simulink model "Simulacao_Exemplo_2B"  (R2020a)
settings: Solver=ode45  StartTime=0.0  StopTime=240  FixedStep=0.1  MaxStep=5e-1  RelTol=1e-3  EnableMultiTasking=on
settings Model: Creator=MeneghettiAir  LastModifiedBy=jhona
settings DataIOCC: LimitDataPoints=on  SaveFormat=Array  ReturnWorkspaceOutputs=off
settings OptimizationCC: LifeSpan=inf
settings DebuggingCC: SolverPrmCheckMsg=warning  SFUnexpectedBacktrackingDiag=warning  SFNoUnconditionalDefaultTransitionDiag=warning  SFExecutionAtInitializationDiag=none  ArithmeticOperatorsInVariantConditions=warning
settings HardwareCC: ProdBitPerPointer=32  ProdBitPerSizeT=32  ProdBitPerPtrDiffT=32  ProdLargestAtomicFloat=None  ProdIntDivRoundTo=Undefined  ProdEndianess=Unspecified  ProdWordSize=32  ProdHWDeviceType=32-bit Generic
settings ModelReferenceCC: PropagateSignalLabelsOutOfModel=off
settings SFSimCC: SimUseLocalCustomCode=off  CustomCodeUndefinedFunction=UseInterfaceOnly
settings RTWCC: RTWUseLocalCustomCode=off
settings CodeAppCC: StateflowObjectComments=on
settings GRTTargetCC: TargetLangStandard=C89/C90 (ANSI)
settings ConfigComp: CovMetricSettings=dw  CovHtmlReporting=on  CovSaveCumulativeToWorkspaceVar=on  CovSaveSingleToWorkspaceVar=on  CovExternalEMLEnable=off  CovSFcnEnable=off

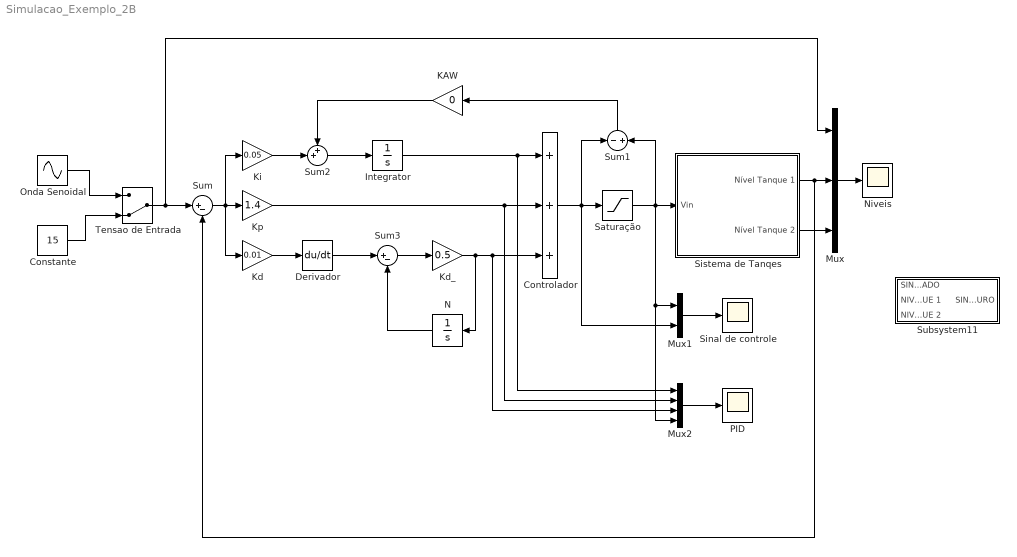
== system Simulacao_Exemplo_2B ==
  Constante : Constant  Value=15
  Controlador : Sum  Inputs=+++
  Derivador : Derivative
  Integrator : Integrator
  KAW : Gain  Gain=0
  Kd : Gain  Gain=0.01
  Kd_ : Gain  Gain=0.5
  Ki : Gain  Gain=0.05
  Kp : Gain  Gain=1.4
  Mux : Mux  Inputs=3
  Mux1 : Mux  Inputs=2
  Mux2 : Mux
  N : Integrator
  Niveis : Scope
  Onda Senoidal : Sin  Amplitude=2  Bias=14  Frequency=0.2  SampleTime=0
  PID : Scope
  Saturação : Saturate  UpperLimit=4  LowerLimit=-4
  Sinal de controle : Scope
  "Sistema de Tanqes " : Subsystem
  Subsystem11 : Subsystem
  Sum : Sum  Inputs=|+-
  Sum1 : Sum  Inputs=-|+
  Sum2 : Sum  Inputs=++|
  Sum3 : Sum  Inputs=|+-
  Tensao de Entrada : ManualSwitch  CurrentSetting=0
  wires:
  "Sistema de Tanqes "/1(Nível Tanque 1) -> Sum/2, Mux/2
  "Sistema de Tanqes "/2(Nível Tanque 2) -> Mux/3
  Mux/1 -> Niveis/1
  Tensao de Entrada/1 -> Sum/1, Mux/1
  Constante/1 -> Tensao de Entrada/2
  Onda Senoidal/1 -> Tensao de Entrada/1
  Mux1/1 -> Sinal de controle/1
  Saturação/1 -> Sum1/2, Mux2/4, Mux1/1, "Sistema de Tanqes "/1(Vin)
  Sum/1 -> Kd/1, Ki/1, Kp/1
  Controlador/1 -> Sum1/1, Saturação/1, Mux1/2
  Integrator/1 -> Mux2/1, Controlador/1
  Kp/1 -> Mux2/2, Controlador/2
  Mux2/1 -> PID/1
  Kd/1 -> Derivador/1
  Sum1/1 -> KAW/1
  KAW/1 -> Sum2/1
  Sum2/1 -> Integrator/1
  Ki/1 -> Sum2/2
  Kd_/1 -> N/1, Mux2/3, Controlador/3
  Sum3/1 -> Kd_/1
  Derivador/1 -> Sum3/1
  N/1 -> Sum3/2

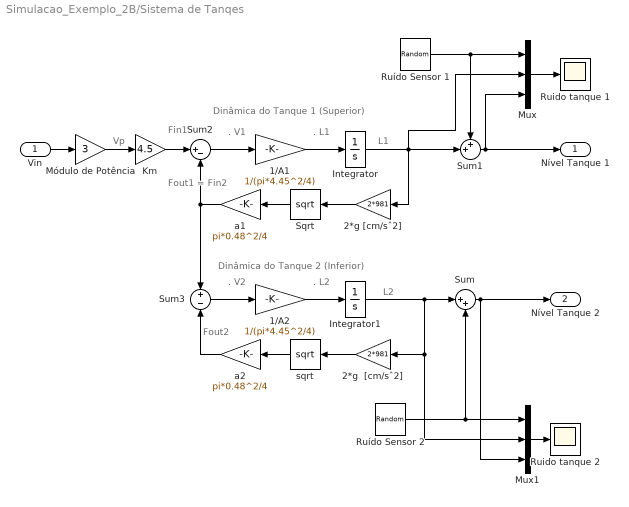
== system Simulacao_Exemplo_2B/Sistema de Tanqes  ==
  note: Dinâmica do Tanque 1 (Superior)
  note: L1
  note: Fin1
  note: Fout1
      | =
      | Fin2
  note: .
      | L1
  note: .
      | V1
  note: L2
  note: Fout2
  note: .
      | L2
  note: .
      | V2
  note: Dinâmica do Tanque 2 (Inferior)
  note: Vp
  Vin : Inport
  1/A1 : Gain  Gain=1/(pi*4.45^2/4)
  1/A2 : Gain  Gain=1/(pi*4.45^2/4)
  2*g  [cm/sˆ2] : Gain  Gain=2*981
  2*g [cm/sˆ2] : Gain  Gain=2*981
  Integrator : Integrator  UpperSaturationLimit=35  LowerSaturationLimit=-2
  Integrator1 : Integrator  UpperSaturationLimit=35  LowerSaturationLimit=-2
  Km : Gain  Gain=4.5
  Mux : Mux  Inputs=3
  Mux1 : Mux  Inputs=3
  Módulo de Potência : Gain  Gain=3
  Ruido tanque 1 : Scope
  Ruido tanque 2 : Scope
  Ruído Sensor 1 : UniformRandomNumber  Minimum=-0.0001  Maximum=0.0001  Seed=round(rand(1)*100)  SampleTime=0.0001
  Ruído Sensor 2 : UniformRandomNumber  Minimum=-0.0001  Maximum=0.0001  Seed=round(rand(1)*100)  SampleTime=0.01
  Sqrt : Sqrt  SaturateOnIntegerOverflow=on
  Sum : Sum  Inputs=|++
  Sum1 : Sum  Inputs=++|
  Sum2 : Sum  Inputs=|+-
  Sum3 : Sum  Inputs=+-
  a1 : Gain  Gain=pi*0.48^2/4
  a2 : Gain  Gain=pi*0.48^2/4
  sqrt : Sqrt  SaturateOnIntegerOverflow=on
  Nível Tanque 1 : Outport
  Nível Tanque 2 : Outport  Port=2
  wires:
  Vin/1 -> Módulo de Potência/1
  Sum/1 -> Nível Tanque 2/1, Mux1/3
  Mux/1 -> Ruido tanque 1/1
  Mux1/1 -> Ruido tanque 2/1
  Sum1/1 -> Nível Tanque 1/1, Mux/3
  Ruído Sensor 1/1 -> Mux/1, Sum1/1
  Ruído Sensor 2/1 -> Sum/2, Mux1/1
  2*g [cm/sˆ2]/1 -> Sqrt/1
  Sqrt/1 -> a1/1
  Km/1 -> Sum2/1
  a1/1 -> Sum2/2, Sum3/1
  Sum2/1 -> 1/A1/1
  1/A1/1 -> Integrator/1
  2*g  [cm/sˆ2]/1 -> sqrt/1
  sqrt/1 -> a2/1
  Sum3/1 -> 1/A2/1
  1/A2/1 -> Integrator1/1
  a2/1 -> Sum3/2
  Módulo de Potência/1 -> Km/1
  Integrator/1 -> Sum1/2, Mux/2, 2*g [cm/sˆ2]/1
  Integrator1/1 -> Mux1/2, 2*g  [cm/sˆ2]/1, Sum/1

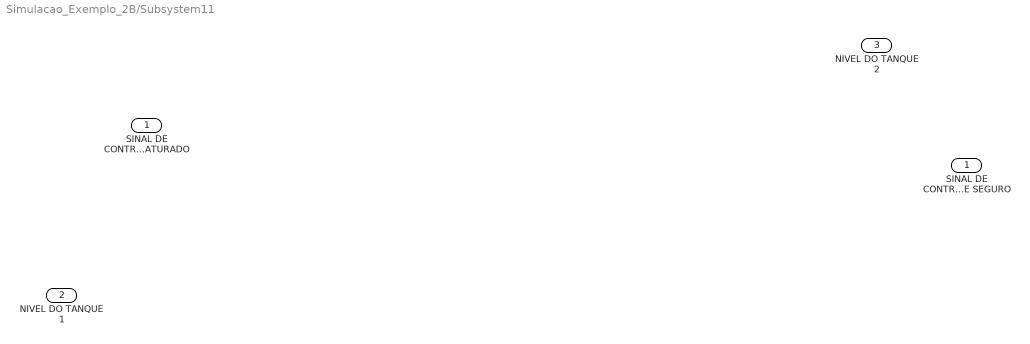
== system Simulacao_Exemplo_2B/Subsystem11 ==
  SINAL DE CONTROLE NÃO SATURADO : Inport
  NIVEL DO TANQUE 1 : Inport  Port=2
  NIVEL DO TANQUE 2 : Inport  Port=3
  SINAL DE CONTROLE SEGURO : Outport
